simulink model "px42LoopCtr20210902"  (R2022a)
settings: Solver=FixedStepDiscrete  StartTime=0.0  StopTime=inf  FixedStep=0.005  RelTol=1e-3  EnableMultiTasking=on
InitFcn:
  | I_x = 0.00478;
  | I_y = 0.00502;
  | I_z = 0.00736;
  | m=1;
  | L=0.11667;
undefined symbols (not defined in the file): dev, DiscIntNeverNeededParam, Main, pwm_output0
libraries: simulink x30, px4lib x3, px4uORBlib x2, sharedtransform x1
(part 2 of 3)

== system px42LoopCtr20210902/Attitude controller/Subsystem6 ==
  roll : Inport
  roll_des : Inport  Port=2
  Add : Sum  Inputs=+----
  Add1 : Sum  Inputs=+-
  Add2 : Sum  Inputs=+-
  Constant1 : Constant  Value=0
  Data Store Read : DataStoreRead  DataStoreName=attitude_flag  IndexOptions=Index vector (dialog)  Indices=1  OutputSizes=1
  Data Store Read1 : DataStoreRead  DataStoreName=roll_speed  IndexOptions=Index vector (dialog)  Indices=1  OutputSizes=1
  Data Store Write : DataStoreWrite  DataStoreName=e_pitch_roll  IndexOptions=Index vector (dialog)  Indices=1  OutputSizes=1
  Demux : Demux  Outputs=3
  Discrete Derivative1 : simulink/Discrete/Discrete Derivative  gainval=1.0  ICPrevScaledInput=0.0  OutMin=[]  OutMax=[]  OutDataType=fixdt(1, 16)  OutScaling=2^-10  DoSatur=off
  Gain : Gain  Gain=0.01/0.0052
  J : Gain  Gain=0.00478
  Mux : Mux  Inputs=3
  Product : Product  Inputs=3
  Product1 : Product
  Sign : Signum
  Slider : SliderBlock  ScaleMax=20
  Slider1 : SliderBlock  ScaleMax=20
  Slider2 : SliderBlock  ScaleMin=2  ScaleMax=10
  Slider3 : SliderBlock  ScaleMax=20
  Slider4 : SliderBlock  ScaleMax=10
  Subsystem1 : Subsystem
  Switch : Switch  Criteria=u2 > Threshold  SaturateOnIntegerOverflow=off  InputSameDT=off
  b : Constant  Value=2.490277777777778
  l : Constant  Value=0.5340277777777778
  u2 : Outport
  wires:
  Data Store Read1/1 -> Mux/3
  Demux/2 -> Add2/2, Subsystem1/2(roll_des)
  Demux/1 -> Add2/1, Subsystem1/1(roll)
  Mux/1 -> Switch/1
  Constant1/1 -> Switch/3
  Switch/1 -> Demux/1
  Data Store Read/1 -> Switch/2
  Add/1 -> J/1
  Gain/1 -> Add/5
  Product1/1 -> Add/4
  Add2/1 -> Add/2, Data Store Write/1
  roll_des/1 -> Mux/2
  Sign/1 -> Product1/1
  Subsystem1/1(v*) -> Discrete Derivative1/1, Add1/2
  Subsystem1/2(H) -> Product/2
  b/1 -> Product/3, Subsystem1/3(b)
  l/1 -> Product1/2
  Discrete Derivative1/1 -> Add/1  "v*_dot"
  roll/1 -> Mux/1
  Demux/3 -> Add1/1, Gain/1  "v"
  Add1/1 -> Product/1, Sign/1  "v-v*"
  Product/1 -> Add/3
  J/1 -> u2/1

== system px42LoopCtr20210902/Attitude controller/Subsystem7 ==
  yaw : Inport
  yaw_des : Inport  Port=2
  Add : Sum  Inputs=+----
  Add1 : Sum  Inputs=+-
  Add2 : Sum  Inputs=+-
  Constant1 : Constant  Value=0
  Data Store Read : DataStoreRead  DataStoreName=attitude_flag  IndexOptions=Index vector (dialog)  Indices=1  OutputSizes=1
  Data Store Read1 : DataStoreRead  DataStoreName=yaw_speed  IndexOptions=Index vector (dialog)  Indices=1  OutputSizes=1
  Data Store Write : DataStoreWrite  DataStoreName=e_pitch_yaw  IndexOptions=Index vector (dialog)  Indices=1  OutputSizes=1
  Demux : Demux  Outputs=3
  Discrete Derivative1 : simulink/Discrete/Discrete Derivative  gainval=1.0  ICPrevScaledInput=0.0  OutMin=[]  OutMax=[]  OutDataType=fixdt(1, 16)  OutScaling=2^-10  DoSatur=off
  Gain : Gain  Gain=0.01/0.0052
  Gain1 : Gain  Gain=0.00502
  Mux : Mux  Inputs=3
  Product : Product  Inputs=3
  Product1 : Product
  Sign : Signum
  Slider : SliderBlock  ScaleMax=20
  Slider1 : SliderBlock  ScaleMax=20
  Slider2 : SliderBlock  ScaleMin=2  ScaleMax=10
  Slider3 : SliderBlock  ScaleMax=20
  Slider4 : SliderBlock  ScaleMax=10
  Subsystem1 : Subsystem
  Switch : Switch  Criteria=u2 > Threshold  SaturateOnIntegerOverflow=off  InputSameDT=off
  b : Constant  Value=2.036184210526316
  l : Constant  Value=0.5282118055555556
  u2 : Outport
  wires:
  Data Store Read1/1 -> Mux/3
  Demux/2 -> Add2/2, Subsystem1/2(pitch_des)
  Demux/1 -> Add2/1, Subsystem1/1(pitch)
  Mux/1 -> Switch/1
  Constant1/1 -> Switch/3
  Switch/1 -> Demux/1
  Data Store Read/1 -> Switch/2
  Gain1/1 -> u2/1
  Gain/1 -> Add/5
  Product1/1 -> Add/4
  Add2/1 -> Add/2, Data Store Write/1
  yaw_des/1 -> Mux/2
  Add/1 -> Gain1/1
  Sign/1 -> Product1/1
  Subsystem1/1(v*) -> Discrete Derivative1/1, Add1/2
  Subsystem1/2(H) -> Product/2
  b/1 -> Product/3, Subsystem1/3(b)
  l/1 -> Product1/2
  Discrete Derivative1/1 -> Add/1  "v*_dot"
  yaw/1 -> Mux/1
  Demux/3 -> Add1/1, Gain/1  "v"
  Add1/1 -> Product/1, Sign/1  "v-v*"
  Product/1 -> Add/3

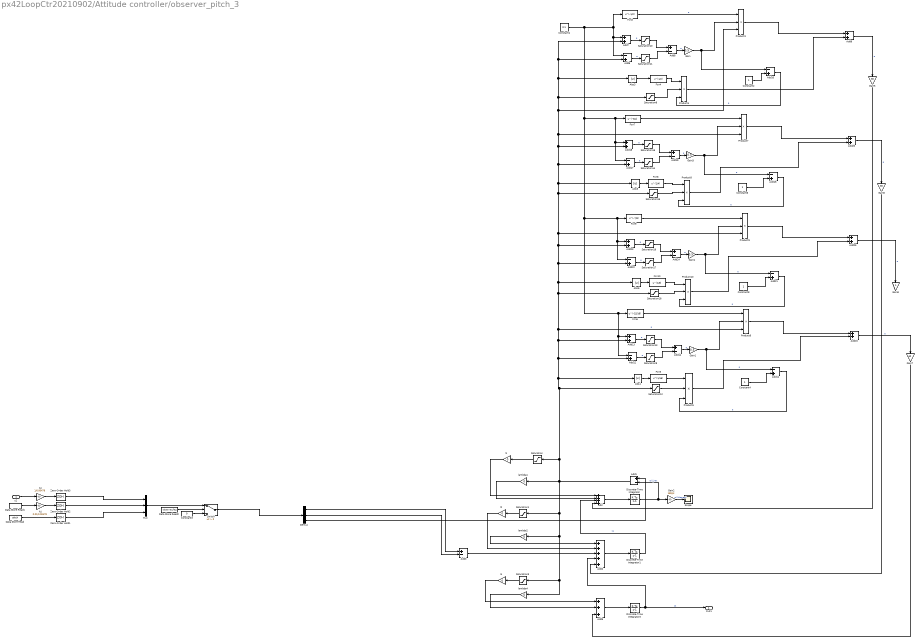
== system px42LoopCtr20210902/Attitude controller/observer_pitch_3 ==
  u2 : Inport
  1/J : Gain  Gain=1/0.00478
  Abs{3..6} (4 alike) : Abs  SaturateOnIntegerOverflow=off
  Add : Sum  Inputs=++++
  Add{1,3,8,14,19,24} (6 alike) : Sum  Inputs=+-
  Add{6,10..12,16..17,21..22} (8 alike) : Sum  Inputs=-+
  Add{7,9,13,15,18,20,23,25} (8 alike) : Sum
  Add2 : Sum  Inputs=+++++
  Add5 : Sum  Inputs=+++
  Constant1 : Constant  Value=0.1
  Constant{2,4,6,8} (4 alike) : Constant
  Constant3 : Constant  Value=0
  Data Store Read : DataStoreRead  DataStoreName=pitch  IndexOptions=Index vector (dialog)  Indices=1  OutputSizes=1
  Data Store Read1 : DataStoreRead  DataStoreName=pitch_speed  IndexOptions=Index vector (dialog)  Indices=1  OutputSizes=1
  Data Store Read2 : DataStoreRead  DataStoreName=observer_flag  IndexOptions=Index vector (dialog)  Indices=1  OutputSizes=1
  Demux : Demux  Outputs=3
  Discrete-Time Integrator : DiscreteIntegrator  SampleTime=-1  ICPrevOutput=DiscIntNeverNeededParam  ICPrevScaledInput=DiscIntNeverNeededParam
  Discrete-Time Integrator1 : DiscreteIntegrator  SampleTime=-1  ICPrevOutput=DiscIntNeverNeededParam  ICPrevScaledInput=DiscIntNeverNeededParam
  Discrete-Time Integrator3 : DiscreteIntegrator  SampleTime=-1  ICPrevOutput=DiscIntNeverNeededParam  ICPrevScaledInput=DiscIntNeverNeededParam
  Fcn10 : Fcn  Expr=u^(1/8)
  Fcn3 : Fcn  Expr=u^(-1/2)
  Fcn4 : Fcn  Expr=u^(1/2)
  Fcn5 : Fcn  Expr=u^(1/16)
  Fcn6 : Fcn  Expr=u^(-15/16)
  Fcn7 : Fcn  Expr=u^(-3/4)
  Fcn8 : Fcn  Expr=u^(1/4)
  Fcn9 : Fcn  Expr=u^(-7/8)
  Gain{,1,3..4} (4 alike) : Gain  Gain=0.5
  Gain2 : Gain  Gain=180/pi
  Gain5 : Gain  Gain=30
  Gain6 : Gain  Gain=30
  Gain7 : Gain  Gain=40
  Gain8 : Gain
  Mux : Mux  Inputs=3
  Product{3..10} (8 alike) : Product  Inputs=3
  Saturation{,1,3,8..19} (15 alike) : Saturate  UpperLimit=1  LowerLimit=-1
  Scope : Scope
  Switch : Switch  Criteria=u2 > Threshold  SaturateOnIntegerOverflow=off  InputSameDT=off
  Zero-Order Hold1 : ZeroOrderHold  SampleTime=-1
  Zero-Order Hold2 : ZeroOrderHold  SampleTime=-1
  Zero-Order Hold3 : ZeroOrderHold  SampleTime=-1
  k/J : Gain  Gain=0.01/0.00478
  l1 : Gain  Gain=0
  l2 : Gain  Gain=0
  l4 : Gain  Gain=0
  lambda1 : Gain  Gain=0
  lambda2 : Gain  Gain=0
  lambda4 : Gain  Gain=0
  Out1 : Outport
  wires:
  Fcn4/1 -> Product4/1
  Fcn3/1 -> Product3/1  "e"
  Gain7/1 -> Add5/3
  Gain6/1 -> Add2/5
  Gain5/1 -> Add/4
  Add9/1 -> Gain5/1  "e"
  Add20/1 -> Gain6/1  "e"
  Add25/1 -> Gain8/1  "e"
  Add15/1 -> Gain7/1  "e"
  Saturation13/1 -> Add14/1
  Add1/1 -> Saturation1/1, lambda2/1, Saturation3/1, lambda4/1, Saturation/1, Saturation15/1, Abs5/1, Add17/2, Add18/2, Abs3/1, Add7/2, Add6/2, Saturation8/1, Product3/3, Product7/3, Product9/3, Add23/2, Add22/2, Abs6/1, Saturation18/1, Product6/3, Add13/2, Add12/2, Abs4/1, Saturation12/1, lambda1/1  "e"
  Add11/1 -> Product5/3  "e"
  Add12/1 -> Saturation9/1  "e"
  Abs4/1 -> Fcn5/1
  Constant4/1 -> Add11/2
  Product6/1 -> Add15/1
  Saturation12/1 -> Product5/2
  Gain1/1 -> Product6/2, Add11/1  "e"
  Add13/1 -> Saturation13/1  "e"
  Fcn6/1 -> Product6/1
  Fcn5/1 -> Product5/1
  Saturation9/1 -> Add14/2
  Product5/1 -> Add15/2
  Constant1/1 -> Fcn9/1, Add23/1, Add22/1, Add13/1, Add12/1, Fcn6/1, Add18/1, Add17/1, Fcn7/1, Add7/1, Add6/1, Fcn3/1
  Add14/1 -> Gain1/1  "e"
  Add24/1 -> Gain4/1  "e"
  Saturation17/1 -> Add24/2
  Product10/1 -> Add25/2
  Fcn10/1 -> Product10/1
  Fcn9/1 -> Product9/1
  Add23/1 -> Saturation19/1  "e"
  Gain4/1 -> Product9/2, Add21/1  "e"
  Saturation18/1 -> Product10/2
  Saturation19/1 -> Add24/1
  Abs6/1 -> Fcn10/1
  Add21/1 -> Product10/3  "e"
  Product9/1 -> Add25/1
  Add22/1 -> Saturation17/1  "e"
  Constant8/1 -> Add21/2
  Product7/1 -> Add20/1
  Saturation15/1 -> Product8/2
  Add17/1 -> Saturation14/1  "e"
  Constant6/1 -> Add16/2
  Gain3/1 -> Product7/2, Add16/1  "e"
  Abs5/1 -> Fcn8/1
  Add16/1 -> Product8/3  "e"
  Saturation16/1 -> Add19/1
  Fcn8/1 -> Product8/1
  Fcn7/1 -> Product7/1
  Product8/1 -> Add20/2
  Add19/1 -> Gain3/1  "e"
  Saturation14/1 -> Add19/2
  Add18/1 -> Saturation16/1  "e"
  Product4/1 -> Add9/2
  Saturation11/1 -> Add8/2
  Saturation10/1 -> Add8/1
  Add10/1 -> Product4/3  "e"
  Constant2/1 -> Add10/2
  Saturation8/1 -> Product4/2
  Abs3/1 -> Fcn4/1
  Product3/1 -> Add9/1
  Gain/1 -> Product3/2, Add10/1
  Add8/1 -> Gain/1  "e"
  Add6/1 -> Saturation11/1  "e"
  Add7/1 -> Saturation10/1  "e"
  Gain2/1 -> Scope/1  "roll(degree)"
  l4/1 -> Add5/1
  lambda4/1 -> Add5/2
  Add5/1 -> Discrete-Time Integrator3/1
  Saturation3/1 -> l4/1
  Add2/1 -> Discrete-Time Integrator1/1
  Add3/1 -> Add2/3
  l2/1 -> Add2/2
  lambda2/1 -> Add2/1
  Saturation1/1 -> l2/1
  Discrete-Time Integrator3/1 -> Out1/1, Add2/4  "z2"
  l1/1 -> Add/1
  Saturation/1 -> l1/1
  lambda1/1 -> Add/2
  Discrete-Time Integrator/1 -> Gain2/1, Add1/2  "roll_hat"
  Discrete-Time Integrator1/1 -> Add/3  "z1"
  Add/1 -> Discrete-Time Integrator/1
  Demux/1 -> Add3/1
  Demux/2 -> Add3/2
  Demux/3 -> Add1/1
  k/J/1 -> Zero-Order Hold2/1
  Data Store Read1/1 -> k/J/1
  Zero-Order Hold2/1 -> Mux/2
  Mux/1 -> Switch/1
  Zero-Order Hold3/1 -> Mux/1
  u2/1 -> 1/J/1
  Switch/1 -> Demux/1
  Data Store Read2/1 -> Switch/2
  Zero-Order Hold1/1 -> Mux/3
  Data Store Read/1 -> Zero-Order Hold1/1
  1/J/1 -> Zero-Order Hold3/1
  Constant3/1 -> Switch/3

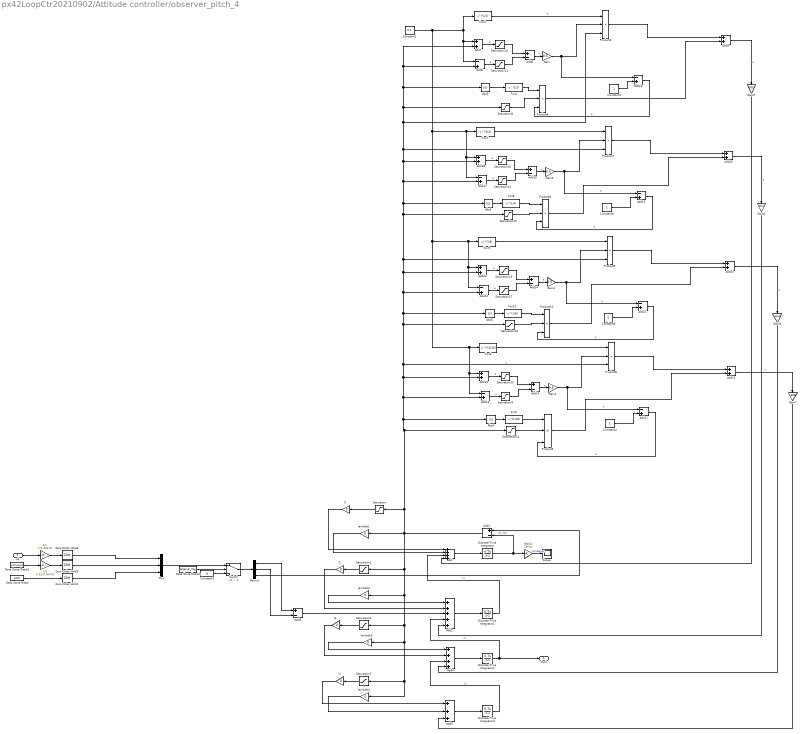
== system px42LoopCtr20210902/Attitude controller/observer_pitch_4 ==
  u2 : Inport
  1/J : Gain  Gain=1/0.00478
  Abs{3..6} (4 alike) : Abs  SaturateOnIntegerOverflow=off
  Add : Sum  Inputs=++++
  Add{1,3,8,14,19,24} (6 alike) : Sum  Inputs=+-
  Add{6,10..12,16..17,21..22} (8 alike) : Sum  Inputs=-+
  Add{7,9,13,15,18,20,23,25} (8 alike) : Sum
  Add2 : Sum  Inputs=+++++
  Add4 : Sum  Inputs=++++
  Add5 : Sum  Inputs=+++
  Constant1 : Constant  Value=0.1
  Constant{2,4,6,8} (4 alike) : Constant
  Constant3 : Constant  Value=0
  Data Store Read : DataStoreRead  DataStoreName=pitch  IndexOptions=Index vector (dialog)  Indices=1  OutputSizes=1
  Data Store Read1 : DataStoreRead  DataStoreName=pitch_speed  IndexOptions=Index vector (dialog)  Indices=1  OutputSizes=1
  Data Store Read2 : DataStoreRead  DataStoreName=observer_flag  IndexOptions=Index vector (dialog)  Indices=1  OutputSizes=1
  Demux : Demux  Outputs=3
  Discrete-Time Integrator{,1..3} (4 alike) : DiscreteIntegrator  SampleTime=-1  ICPrevOutput=DiscIntNeverNeededParam  ICPrevScaledInput=DiscIntNeverNeededParam
  Fcn10 : Fcn  Expr=u^(1/8)
  Fcn3 : Fcn  Expr=u^(-1/2)
  Fcn4 : Fcn  Expr=u^(1/2)
  Fcn5 : Fcn  Expr=u^(1/16)
  Fcn6 : Fcn  Expr=u^(-15/16)
  Fcn7 : Fcn  Expr=u^(-3/4)
  Fcn8 : Fcn  Expr=u^(1/4)
  Fcn9 : Fcn  Expr=u^(-7/8)
  Gain{,1,3..4} (4 alike) : Gain  Gain=0.5
  Gain2 : Gain  Gain=180/pi
  Gain5 : Gain  Gain=300
  Gain6 : Gain  Gain=3000
  Gain7 : Gain  Gain=300
  Gain8 : Gain  Gain=5000
  Mux : Mux  Inputs=3
  Product{3..10} (8 alike) : Product  Inputs=3
  Saturation{,1..3,8..19} (16 alike) : Saturate  UpperLimit=1  LowerLimit=-1
  Scope : Scope
  Switch : Switch  Criteria=u2 > Threshold  SaturateOnIntegerOverflow=off  InputSameDT=off
  Zero-Order Hold1 : ZeroOrderHold  SampleTime=-1
  Zero-Order Hold2 : ZeroOrderHold  SampleTime=-1
  Zero-Order Hold3 : ZeroOrderHold  SampleTime=-1
  k/J : Gain  Gain=0.01/0.00478
  l{1..4} (4 alike) : Gain  Gain=0
  lambda{1..4} (4 alike) : Gain  Gain=0
  Out1 : Outport
  wires:
  Zero-Order Hold1/1 -> Mux/3
  Demux/3 -> Add1/1
  Demux/2 -> Add3/2
  Demux/1 -> Add3/1
  Zero-Order Hold3/1 -> Mux/1
  Mux/1 -> Switch/1
  Constant3/1 -> Switch/3
  Zero-Order Hold2/1 -> Mux/2
  Switch/1 -> Demux/1
  Add/1 -> Discrete-Time Integrator/1
  Discrete-Time Integrator1/1 -> Add/3  "z1"
  Discrete-Time Integrator/1 -> Add1/2, Gain2/1  "roll_hat"
  Data Store Read/1 -> Zero-Order Hold1/1
  lambda1/1 -> Add/2
  Saturation/1 -> l1/1
  l1/1 -> Add/1
  Discrete-Time Integrator2/1 -> Out1/1, Add2/4  "z2"
  Saturation1/1 -> l2/1
  lambda2/1 -> Add2/1
  l2/1 -> Add2/2
  Data Store Read1/1 -> k/J/1
  k/J/1 -> Zero-Order Hold2/1
  u2/1 -> 1/J/1
  1/J/1 -> Zero-Order Hold3/1
  Add3/1 -> Add2/3
  Add2/1 -> Discrete-Time Integrator1/1
  Discrete-Time Integrator3/1 -> Add4/3  "z3"
  Add4/1 -> Discrete-Time Integrator2/1
  Saturation2/1 -> l3/1
  lambda3/1 -> Add4/1
  l3/1 -> Add4/2
  Saturation3/1 -> l4/1
  Add5/1 -> Discrete-Time Integrator3/1
  lambda4/1 -> Add5/2
  l4/1 -> Add5/1
  Gain2/1 -> Scope/1  "roll(degree)"
  Add7/1 -> Saturation10/1  "e"
  Add6/1 -> Saturation11/1  "e"
  Add8/1 -> Gain/1  "e"
  Gain/1 -> Add10/1, Product3/2
  Product3/1 -> Add9/1
  Abs3/1 -> Fcn4/1
  Saturation8/1 -> Product4/2
  Constant2/1 -> Add10/2
  Add10/1 -> Product4/3  "e"
  Saturation10/1 -> Add8/1
  Saturation11/1 -> Add8/2
  Product4/1 -> Add9/2
  Add18/1 -> Saturation16/1  "e"
  Saturation14/1 -> Add19/2
  Add19/1 -> Gain3/1  "e"
  Product8/1 -> Add20/2
  Fcn7/1 -> Product7/1
  Fcn8/1 -> Product8/1
  Saturation16/1 -> Add19/1
  Add16/1 -> Product8/3  "e"
  Abs5/1 -> Fcn8/1
  Gain3/1 -> Add16/1, Product7/2  "e"
  Constant6/1 -> Add16/2
  Add17/1 -> Saturation14/1  "e"
  Saturation15/1 -> Product8/2
  Product7/1 -> Add20/1
  Constant8/1 -> Add21/2
  Add22/1 -> Saturation17/1  "e"
  Product9/1 -> Add25/1
  Add21/1 -> Product10/3  "e"
  Abs6/1 -> Fcn10/1
  Saturation19/1 -> Add24/1
  Saturation18/1 -> Product10/2
  Gain4/1 -> Add21/1, Product9/2  "e"
  Add23/1 -> Saturation19/1  "e"
  Fcn9/1 -> Product9/1
  Fcn10/1 -> Product10/1
  Product10/1 -> Add25/2
  Saturation17/1 -> Add24/2
  Add24/1 -> Gain4/1  "e"
  Add14/1 -> Gain1/1  "e"
  Constant1/1 -> Fcn3/1, Add6/1, Add7/1, Fcn7/1, Add17/1, Add18/1, Fcn6/1, Add12/1, Add13/1, Add22/1, Add23/1, Fcn9/1
  Product5/1 -> Add15/2
  Saturation9/1 -> Add14/2
  Fcn5/1 -> Product5/1
  Fcn6/1 -> Product6/1
  Add13/1 -> Saturation13/1  "e"
  Gain1/1 -> Add11/1, Product6/2  "e"
  Saturation12/1 -> Product5/2
  Product6/1 -> Add15/1
  Constant4/1 -> Add11/2
  Abs4/1 -> Fcn5/1
  Add12/1 -> Saturation9/1  "e"
  Add11/1 -> Product5/3  "e"
  Add1/1 -> lambda1/1, Saturation12/1, Abs4/1, Add12/2, Add13/2, Product6/3, Saturation18/1, Abs6/1, Add22/2, Add23/2, Product9/3, Product7/3, Product3/3, Saturation8/1, Add6/2, Add7/2, Abs3/1, Add18/2, Add17/2, Abs5/1, Saturation15/1, Saturation/1, lambda4/1, Saturation3/1, lambda3/1, Saturation2/1, lambda2/1, Saturation1/1  "e"
  Saturation13/1 -> Add14/1
  Add15/1 -> Gain7/1  "e"
  Add25/1 -> Gain8/1  "e"
  Add20/1 -> Gain6/1  "e"
  Add9/1 -> Gain5/1  "e"
  Gain5/1 -> Add/4
  Gain6/1 -> Add2/5
  Gain7/1 -> Add5/3
  Gain8/1 -> Add4/4
  Fcn3/1 -> Product3/1  "e"
  Fcn4/1 -> Product4/1
  Data Store Read2/1 -> Switch/2

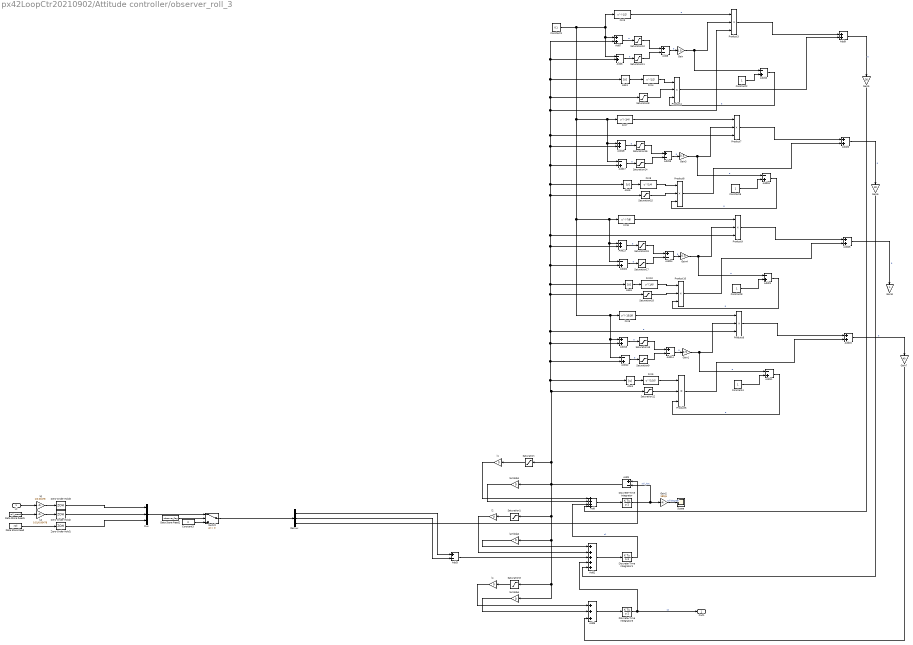
== system px42LoopCtr20210902/Attitude controller/observer_roll_3 ==
  u2 : Inport
  1/J : Gain  Gain=1/0.00478
  Abs{3..6} (4 alike) : Abs  SaturateOnIntegerOverflow=off
  Add : Sum  Inputs=++++
  Add{1,3,8,14,19,24} (6 alike) : Sum  Inputs=+-
  Add{6,10..12,16..17,21..22} (8 alike) : Sum  Inputs=-+
  Add{7,9,13,15,18,20,23,25} (8 alike) : Sum
  Add2 : Sum  Inputs=+++++
  Add5 : Sum  Inputs=+++
  Constant1 : Constant  Value=0.1
  Constant{2,4,6,8} (4 alike) : Constant
  Constant3 : Constant  Value=0
  Data Store Read : DataStoreRead  DataStoreName=roll  IndexOptions=Index vector (dialog)  Indices=1  OutputSizes=1
  Data Store Read1 : DataStoreRead  DataStoreName=roll_speed  IndexOptions=Index vector (dialog)  Indices=1  OutputSizes=1
  Data Store Read2 : DataStoreRead  DataStoreName=observer_flag  IndexOptions=Index vector (dialog)  Indices=1  OutputSizes=1
  Demux : Demux  Outputs=3
  Discrete-Time Integrator : DiscreteIntegrator  SampleTime=-1  ICPrevOutput=DiscIntNeverNeededParam  ICPrevScaledInput=DiscIntNeverNeededParam
  Discrete-Time Integrator1 : DiscreteIntegrator  SampleTime=-1  ICPrevOutput=DiscIntNeverNeededParam  ICPrevScaledInput=DiscIntNeverNeededParam
  Discrete-Time Integrator3 : DiscreteIntegrator  SampleTime=-1  ICPrevOutput=DiscIntNeverNeededParam  ICPrevScaledInput=DiscIntNeverNeededParam
  Fcn10 : Fcn  Expr=u^(1/8)
  Fcn3 : Fcn  Expr=u^(-1/2)
  Fcn4 : Fcn  Expr=u^(1/2)
  Fcn5 : Fcn  Expr=u^(1/16)
  Fcn6 : Fcn  Expr=u^(-15/16)
  Fcn7 : Fcn  Expr=u^(-3/4)
  Fcn8 : Fcn  Expr=u^(1/4)
  Fcn9 : Fcn  Expr=u^(-7/8)
  Gain{,1,3..4} (4 alike) : Gain  Gain=0.5
  Gain2 : Gain  Gain=180/pi
  Gain5 : Gain  Gain=30
  Gain6 : Gain  Gain=30
  Gain7 : Gain  Gain=40
  Gain8 : Gain
  Mux : Mux  Inputs=3
  Product{3..10} (8 alike) : Product  Inputs=3
  Saturation{,1,3,8..19} (15 alike) : Saturate  UpperLimit=1  LowerLimit=-1
  Scope : Scope
  Switch : Switch  Criteria=u2 > Threshold  SaturateOnIntegerOverflow=off  InputSameDT=off
  Zero-Order Hold1 : ZeroOrderHold  SampleTime=-1
  Zero-Order Hold2 : ZeroOrderHold  SampleTime=-1
  Zero-Order Hold3 : ZeroOrderHold  SampleTime=-1
  k/J : Gain  Gain=0.01/0.00478
  l1 : Gain  Gain=0
  l2 : Gain  Gain=0
  l4 : Gain  Gain=0
  lambda1 : Gain  Gain=0
  lambda2 : Gain  Gain=0
  lambda4 : Gain  Gain=0
  Out1 : Outport
  wires:
  Demux/3 -> Add1/1
  Demux/2 -> Add3/2
  Demux/1 -> Add3/1
  Add/1 -> Discrete-Time Integrator/1
  Discrete-Time Integrator1/1 -> Add/3  "z1"
  Discrete-Time Integrator/1 -> Add1/2, Gain2/1  "roll_hat"
  lambda1/1 -> Add/2
  Saturation/1 -> l1/1
  l1/1 -> Add/1
  Discrete-Time Integrator3/1 -> Add2/4, Out1/1  "z2"
  Saturation1/1 -> l2/1
  lambda2/1 -> Add2/1
  l2/1 -> Add2/2
  Add3/1 -> Add2/3
  Add2/1 -> Discrete-Time Integrator1/1
  Saturation3/1 -> l4/1
  Add5/1 -> Discrete-Time Integrator3/1
  lambda4/1 -> Add5/2
  l4/1 -> Add5/1
  Gain2/1 -> Scope/1  "roll(degree)"
  Add7/1 -> Saturation10/1  "e"
  Add6/1 -> Saturation11/1  "e"
  Add8/1 -> Gain/1  "e"
  Gain/1 -> Add10/1, Product3/2
  Product3/1 -> Add9/1
  Abs3/1 -> Fcn4/1
  Saturation8/1 -> Product4/2
  Constant2/1 -> Add10/2
  Add10/1 -> Product4/3  "e"
  Saturation10/1 -> Add8/1
  Saturation11/1 -> Add8/2
  Product4/1 -> Add9/2
  Add18/1 -> Saturation16/1  "e"
  Saturation14/1 -> Add19/2
  Add19/1 -> Gain3/1  "e"
  Product8/1 -> Add20/2
  Fcn7/1 -> Product7/1
  Fcn8/1 -> Product8/1
  Saturation16/1 -> Add19/1
  Add16/1 -> Product8/3  "e"
  Abs5/1 -> Fcn8/1
  Gain3/1 -> Add16/1, Product7/2  "e"
  Constant6/1 -> Add16/2
  Add17/1 -> Saturation14/1  "e"
  Saturation15/1 -> Product8/2
  Product7/1 -> Add20/1
  Constant8/1 -> Add21/2
  Add22/1 -> Saturation17/1  "e"
  Product9/1 -> Add25/1
  Add21/1 -> Product10/3  "e"
  Abs6/1 -> Fcn10/1
  Saturation19/1 -> Add24/1
  Saturation18/1 -> Product10/2
  Gain4/1 -> Add21/1, Product9/2  "e"
  Add23/1 -> Saturation19/1  "e"
  Fcn9/1 -> Product9/1
  Fcn10/1 -> Product10/1
  Product10/1 -> Add25/2
  Saturation17/1 -> Add24/2
  Add24/1 -> Gain4/1  "e"
  Add14/1 -> Gain1/1  "e"
  Constant1/1 -> Fcn3/1, Add6/1, Add7/1, Fcn7/1, Add17/1, Add18/1, Fcn6/1, Add12/1, Add13/1, Add22/1, Add23/1, Fcn9/1
  Product5/1 -> Add15/2
  Saturation9/1 -> Add14/2
  Fcn5/1 -> Product5/1
  Fcn6/1 -> Product6/1
  Add13/1 -> Saturation13/1  "e"
  Gain1/1 -> Add11/1, Product6/2  "e"
  Saturation12/1 -> Product5/2
  Product6/1 -> Add15/1
  Constant4/1 -> Add11/2
  Abs4/1 -> Fcn5/1
  Add12/1 -> Saturation9/1  "e"
  Add11/1 -> Product5/3  "e"
  Add1/1 -> lambda1/1, Saturation12/1, Abs4/1, Add12/2, Add13/2, Product6/3, Saturation18/1, Abs6/1, Add22/2, Add23/2, Product9/3, Product7/3, Product3/3, Saturation8/1, Add6/2, Add7/2, Abs3/1, Add18/2, Add17/2, Abs5/1, Saturation15/1, Saturation/1, lambda4/1, Saturation3/1, lambda2/1, Saturation1/1  "e"
  Saturation13/1 -> Add14/1
  Add15/1 -> Gain7/1  "e"
  Add25/1 -> Gain8/1  "e"
  Add20/1 -> Gain6/1  "e"
  Add9/1 -> Gain5/1  "e"
  Gain5/1 -> Add/4
  Gain6/1 -> Add2/5
  Gain7/1 -> Add5/3
  Fcn3/1 -> Product3/1  "e"
  Fcn4/1 -> Product4/1
  Constant3/1 -> Switch/3
  u2/1 -> 1/J/1
  Zero-Order Hold1/1 -> Mux/3
  Zero-Order Hold2/1 -> Mux/2
  Zero-Order Hold3/1 -> Mux/1
  Data Store Read/1 -> Zero-Order Hold1/1
  Switch/1 -> Demux/1
  Data Store Read2/1 -> Switch/2
  Data Store Read1/1 -> k/J/1
  1/J/1 -> Zero-Order Hold3/1
  Mux/1 -> Switch/1
  k/J/1 -> Zero-Order Hold2/1

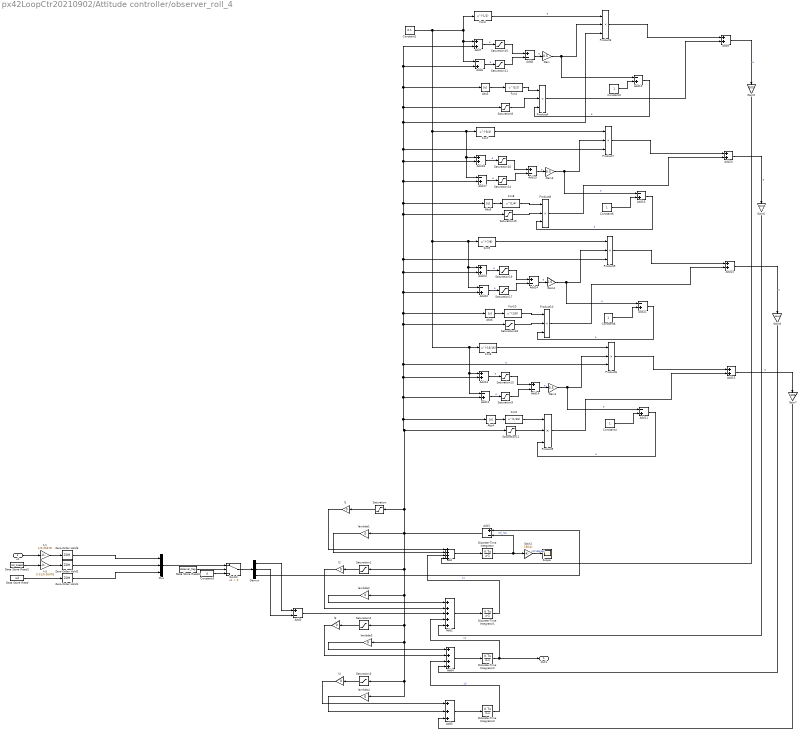
== system px42LoopCtr20210902/Attitude controller/observer_roll_4 ==
  u2 : Inport
  1/J : Gain  Gain=1/0.00478
  Abs{3..6} (4 alike) : Abs  SaturateOnIntegerOverflow=off
  Add : Sum  Inputs=++++
  Add{1,3,8,14,19,24} (6 alike) : Sum  Inputs=+-
  Add{6,10..12,16..17,21..22} (8 alike) : Sum  Inputs=-+
  Add{7,9,13,15,18,20,23,25} (8 alike) : Sum
  Add2 : Sum  Inputs=+++++
  Add4 : Sum  Inputs=++++
  Add5 : Sum  Inputs=+++
  Constant1 : Constant  Value=0.1
  Constant{2,4,6,8} (4 alike) : Constant
  Constant3 : Constant  Value=0
  Data Store Read : DataStoreRead  DataStoreName=roll  IndexOptions=Index vector (dialog)  Indices=1  OutputSizes=1
  Data Store Read1 : DataStoreRead  DataStoreName=roll_speed  IndexOptions=Index vector (dialog)  Indices=1  OutputSizes=1
  Data Store Read2 : DataStoreRead  DataStoreName=observer_flag  IndexOptions=Index vector (dialog)  Indices=1  OutputSizes=1
  Demux : Demux  Outputs=3
  Discrete-Time Integrator{,1..3} (4 alike) : DiscreteIntegrator  SampleTime=-1  ICPrevOutput=DiscIntNeverNeededParam  ICPrevScaledInput=DiscIntNeverNeededParam
  Fcn10 : Fcn  Expr=u^(1/8)
  Fcn3 : Fcn  Expr=u^(-1/2)
  Fcn4 : Fcn  Expr=u^(1/2)
  Fcn5 : Fcn  Expr=u^(1/16)
  Fcn6 : Fcn  Expr=u^(-15/16)
  Fcn7 : Fcn  Expr=u^(-3/4)
  Fcn8 : Fcn  Expr=u^(1/4)
  Fcn9 : Fcn  Expr=u^(-7/8)
  Gain{,1,3..4} (4 alike) : Gain  Gain=0.5
  Gain2 : Gain  Gain=180/pi
  Gain5 : Gain  Gain=300
  Gain6 : Gain  Gain=3000
  Gain7 : Gain  Gain=300
  Gain8 : Gain  Gain=5000
  Mux : Mux  Inputs=3
  Product{3..10} (8 alike) : Product  Inputs=3
  Saturation{,1..3,8..19} (16 alike) : Saturate  UpperLimit=1  LowerLimit=-1
  Scope : Scope
  Switch : Switch  Criteria=u2 > Threshold  SaturateOnIntegerOverflow=off  InputSameDT=off
  Zero-Order Hold1 : ZeroOrderHold  SampleTime=-1
  Zero-Order Hold2 : ZeroOrderHold  SampleTime=-1
  Zero-Order Hold3 : ZeroOrderHold  SampleTime=-1
  k/J : Gain  Gain=0.01/0.00478
  l{1..4} (4 alike) : Gain  Gain=0
  lambda{1..4} (4 alike) : Gain  Gain=0
  Out1 : Outport
  wires:
  Fcn4/1 -> Product4/1
  Fcn3/1 -> Product3/1  "e"
  Gain8/1 -> Add4/4
  Gain7/1 -> Add5/3
  Gain6/1 -> Add2/5
  Gain5/1 -> Add/4
  Add9/1 -> Gain5/1  "e"
  Add20/1 -> Gain6/1  "e"
  Add25/1 -> Gain8/1  "e"
  Add15/1 -> Gain7/1  "e"
  Saturation13/1 -> Add14/1
  Add1/1 -> Saturation1/1, lambda2/1, Saturation2/1, lambda3/1, Saturation3/1, lambda4/1, Saturation/1, Saturation15/1, Abs5/1, Add17/2, Add18/2, Abs3/1, Add7/2, Add6/2, Saturation8/1, Product3/3, Product7/3, Product9/3, Add23/2, Add22/2, Abs6/1, Saturation18/1, Product6/3, Add13/2, Add12/2, Abs4/1, Saturation12/1, lambda1/1  "e"
  Add11/1 -> Product5/3  "e"
  Add12/1 -> Saturation9/1  "e"
  Abs4/1 -> Fcn5/1
  Constant4/1 -> Add11/2
  Product6/1 -> Add15/1
  Saturation12/1 -> Product5/2
  Gain1/1 -> Product6/2, Add11/1  "e"
  Add13/1 -> Saturation13/1  "e"
  Fcn6/1 -> Product6/1
  Fcn5/1 -> Product5/1
  Saturation9/1 -> Add14/2
  Product5/1 -> Add15/2
  Constant1/1 -> Fcn9/1, Add23/1, Add22/1, Add13/1, Add12/1, Fcn6/1, Add18/1, Add17/1, Fcn7/1, Add7/1, Add6/1, Fcn3/1
  Add14/1 -> Gain1/1  "e"
  Add24/1 -> Gain4/1  "e"
  Saturation17/1 -> Add24/2
  Product10/1 -> Add25/2
  Fcn10/1 -> Product10/1
  Fcn9/1 -> Product9/1
  Add23/1 -> Saturation19/1  "e"
  Gain4/1 -> Product9/2, Add21/1  "e"
  Saturation18/1 -> Product10/2
  Saturation19/1 -> Add24/1
  Abs6/1 -> Fcn10/1
  Add21/1 -> Product10/3  "e"
  Product9/1 -> Add25/1
  Add22/1 -> Saturation17/1  "e"
  Constant8/1 -> Add21/2
  Product7/1 -> Add20/1
  Saturation15/1 -> Product8/2
  Add17/1 -> Saturation14/1  "e"
  Constant6/1 -> Add16/2
  Gain3/1 -> Product7/2, Add16/1  "e"
  Abs5/1 -> Fcn8/1
  Add16/1 -> Product8/3  "e"
  Saturation16/1 -> Add19/1
  Fcn8/1 -> Product8/1
  Fcn7/1 -> Product7/1
  Product8/1 -> Add20/2
  Add19/1 -> Gain3/1  "e"
  Saturation14/1 -> Add19/2
  Add18/1 -> Saturation16/1  "e"
  Product4/1 -> Add9/2
  Saturation11/1 -> Add8/2
  Saturation10/1 -> Add8/1
  Add10/1 -> Product4/3  "e"
  Constant2/1 -> Add10/2
  Saturation8/1 -> Product4/2
  Abs3/1 -> Fcn4/1
  Product3/1 -> Add9/1
  Gain/1 -> Product3/2, Add10/1
  Add8/1 -> Gain/1  "e"
  Add6/1 -> Saturation11/1  "e"
  Add7/1 -> Saturation10/1  "e"
  Gain2/1 -> Scope/1  "roll(degree)"
  l4/1 -> Add5/1
  lambda4/1 -> Add5/2
  Add5/1 -> Discrete-Time Integrator3/1
  Saturation3/1 -> l4/1
  l3/1 -> Add4/2
  lambda3/1 -> Add4/1
  Saturation2/1 -> l3/1
  Add4/1 -> Discrete-Time Integrator2/1
  Discrete-Time Integrator3/1 -> Add4/3  "z3"
  Add2/1 -> Discrete-Time Integrator1/1
  Add3/1 -> Add2/3
  1/J/1 -> Zero-Order Hold3/1
  u2/1 -> 1/J/1
  k/J/1 -> Zero-Order Hold2/1
  Data Store Read1/1 -> k/J/1
  l2/1 -> Add2/2
  lambda2/1 -> Add2/1
  Saturation1/1 -> l2/1
  Discrete-Time Integrator2/1 -> Add2/4, Out1/1  "z2"
  l1/1 -> Add/1
  Saturation/1 -> l1/1
  lambda1/1 -> Add/2
  Data Store Read/1 -> Zero-Order Hold1/1
  Discrete-Time Integrator/1 -> Gain2/1, Add1/2  "roll_hat"
  Discrete-Time Integrator1/1 -> Add/3  "z1"
  Add/1 -> Discrete-Time Integrator/1
  Switch/1 -> Demux/1
  Zero-Order Hold2/1 -> Mux/2
  Data Store Read2/1 -> Switch/2
  Constant3/1 -> Switch/3
  Mux/1 -> Switch/1
  Zero-Order Hold3/1 -> Mux/1
  Demux/1 -> Add3/1
  Demux/2 -> Add3/2
  Demux/3 -> Add1/1
  Zero-Order Hold1/1 -> Mux/3

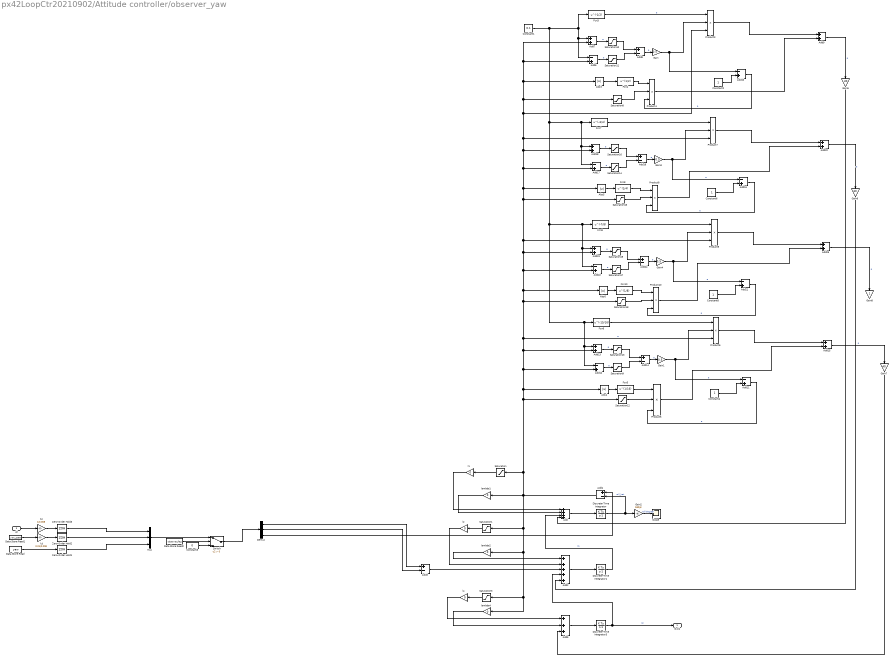
== system px42LoopCtr20210902/Attitude controller/observer_yaw ==
  u2 : Inport
  1/J : Gain  Gain=1/0.008
  Abs{3..6} (4 alike) : Abs  SaturateOnIntegerOverflow=off
  Add : Sum  Inputs=++++
  Add{1,3,8,14,19,24} (6 alike) : Sum  Inputs=+-
  Add{6,10..12,16..17,21..22} (8 alike) : Sum  Inputs=-+
  Add{7,9,13,15,18,20,23,25} (8 alike) : Sum
  Add2 : Sum  Inputs=+++++
  Add5 : Sum  Inputs=+++
  Constant1 : Constant  Value=0.1
  Constant{2,4,6,8} (4 alike) : Constant
  Constant3 : Constant  Value=0
  Data Store Read : DataStoreRead  DataStoreName=yaw  IndexOptions=Index vector (dialog)  Indices=1  OutputSizes=1
  Data Store Read1 : DataStoreRead  DataStoreName=yaw_speed  IndexOptions=Index vector (dialog)  Indices=1  OutputSizes=1
  Data Store Read2 : DataStoreRead  DataStoreName=observer_flag  IndexOptions=Index vector (dialog)  Indices=1  OutputSizes=1
  Demux : Demux  Outputs=3
  Discrete-Time Integrator : DiscreteIntegrator  SampleTime=-1  ICPrevOutput=DiscIntNeverNeededParam  ICPrevScaledInput=DiscIntNeverNeededParam
  Discrete-Time Integrator1 : DiscreteIntegrator  SampleTime=-1  ICPrevOutput=DiscIntNeverNeededParam  ICPrevScaledInput=DiscIntNeverNeededParam
  Discrete-Time Integrator3 : DiscreteIntegrator  SampleTime=-1  ICPrevOutput=DiscIntNeverNeededParam  ICPrevScaledInput=DiscIntNeverNeededParam
  Fcn10 : Fcn  Expr=u^(1/8)
  Fcn3 : Fcn  Expr=u^(-1/2)
  Fcn4 : Fcn  Expr=u^(1/2)
  Fcn5 : Fcn  Expr=u^(1/16)
  Fcn6 : Fcn  Expr=u^(-15/16)
  Fcn7 : Fcn  Expr=u^(-3/4)
  Fcn8 : Fcn  Expr=u^(1/4)
  Fcn9 : Fcn  Expr=u^(-7/8)
  Gain{,1,3..4} (4 alike) : Gain  Gain=0.5
  Gain2 : Gain  Gain=180/pi
  Gain5 : Gain  Gain=30
  Gain6 : Gain  Gain=30
  Gain7 : Gain  Gain=40
  Gain8 : Gain
  Mux : Mux  Inputs=3
  Product{3..10} (8 alike) : Product  Inputs=3
  Saturation{,1,3,8..19} (15 alike) : Saturate  UpperLimit=1  LowerLimit=-1
  Scope : Scope
  Switch : Switch  Criteria=u2 > Threshold  SaturateOnIntegerOverflow=off  InputSameDT=off
  Zero-Order Hold1 : ZeroOrderHold  SampleTime=-1
  Zero-Order Hold2 : ZeroOrderHold  SampleTime=-1
  Zero-Order Hold3 : ZeroOrderHold  SampleTime=-1
  k/J : Gain  Gain=0.01/0.008
  l1 : Gain  Gain=0
  l2 : Gain  Gain=0
  l4 : Gain  Gain=0
  lambda1 : Gain  Gain=0
  lambda2 : Gain  Gain=0
  lambda4 : Gain  Gain=0
  Out1 : Outport
  wires:
  Fcn4/1 -> Product4/1
  Fcn3/1 -> Product3/1  "e"
  Gain7/1 -> Add5/3
  Gain6/1 -> Add2/5
  Gain5/1 -> Add/4
  Add9/1 -> Gain5/1  "e"
  Add20/1 -> Gain6/1  "e"
  Add25/1 -> Gain8/1  "e"
  Add15/1 -> Gain7/1  "e"
  Saturation13/1 -> Add14/1
  Add1/1 -> Saturation1/1, lambda2/1, Saturation3/1, lambda4/1, Saturation/1, Saturation15/1, Abs5/1, Add17/2, Add18/2, Abs3/1, Add7/2, Add6/2, Saturation8/1, Product3/3, Product7/3, Product9/3, Add23/2, Add22/2, Abs6/1, Saturation18/1, Product6/3, Add13/2, Add12/2, Abs4/1, Saturation12/1, lambda1/1  "e"
  Add11/1 -> Product5/3  "e"
  Add12/1 -> Saturation9/1  "e"
  Abs4/1 -> Fcn5/1
  Constant4/1 -> Add11/2
  Product6/1 -> Add15/1
  Saturation12/1 -> Product5/2
  Gain1/1 -> Product6/2, Add11/1  "e"
  Add13/1 -> Saturation13/1  "e"
  Fcn6/1 -> Product6/1
  Fcn5/1 -> Product5/1
  Saturation9/1 -> Add14/2
  Product5/1 -> Add15/2
  Constant1/1 -> Fcn9/1, Add23/1, Add22/1, Add13/1, Add12/1, Fcn6/1, Add18/1, Add17/1, Fcn7/1, Add7/1, Add6/1, Fcn3/1
  Add14/1 -> Gain1/1  "e"
  Add24/1 -> Gain4/1  "e"
  Saturation17/1 -> Add24/2
  Product10/1 -> Add25/2
  Fcn10/1 -> Product10/1
  Fcn9/1 -> Product9/1
  Add23/1 -> Saturation19/1  "e"
  Gain4/1 -> Product9/2, Add21/1  "e"
  Saturation18/1 -> Product10/2
  Saturation19/1 -> Add24/1
  Abs6/1 -> Fcn10/1
  Add21/1 -> Product10/3  "e"
  Product9/1 -> Add25/1
  Add22/1 -> Saturation17/1  "e"
  Constant8/1 -> Add21/2
  Product7/1 -> Add20/1
  Saturation15/1 -> Product8/2
  Add17/1 -> Saturation14/1  "e"
  Constant6/1 -> Add16/2
  Gain3/1 -> Product7/2, Add16/1  "e"
  Abs5/1 -> Fcn8/1
  Add16/1 -> Product8/3  "e"
  Saturation16/1 -> Add19/1
  Fcn8/1 -> Product8/1
  Fcn7/1 -> Product7/1
  Product8/1 -> Add20/2
  Add19/1 -> Gain3/1  "e"
  Saturation14/1 -> Add19/2
  Add18/1 -> Saturation16/1  "e"
  Product4/1 -> Add9/2
  Saturation11/1 -> Add8/2
  Saturation10/1 -> Add8/1
  Add10/1 -> Product4/3  "e"
  Constant2/1 -> Add10/2
  Saturation8/1 -> Product4/2
  Abs3/1 -> Fcn4/1
  Product3/1 -> Add9/1
  Gain/1 -> Product3/2, Add10/1
  Add8/1 -> Gain/1  "e"
  Add6/1 -> Saturation11/1  "e"
  Add7/1 -> Saturation10/1  "e"
  Gain2/1 -> Scope/1  "roll(degree)"
  l4/1 -> Add5/1
  lambda4/1 -> Add5/2
  Add5/1 -> Discrete-Time Integrator3/1
  Saturation3/1 -> l4/1
  Add2/1 -> Discrete-Time Integrator1/1
  Add3/1 -> Add2/3
  l2/1 -> Add2/2
  lambda2/1 -> Add2/1
  Saturation1/1 -> l2/1
  Discrete-Time Integrator3/1 -> Out1/1, Add2/4  "z2"
  l1/1 -> Add/1
  Saturation/1 -> l1/1
  lambda1/1 -> Add/2
  Discrete-Time Integrator/1 -> Gain2/1, Add1/2  "roll_hat"
  Discrete-Time Integrator1/1 -> Add/3  "z1"
  Add/1 -> Discrete-Time Integrator/1
  Demux/1 -> Add3/1
  Demux/2 -> Add3/2
  Demux/3 -> Add1/1
  k/J/1 -> Zero-Order Hold2/1
  Zero-Order Hold1/1 -> Mux/3
  Data Store Read/1 -> Zero-Order Hold1/1
  Constant3/1 -> Switch/3
  Data Store Read2/1 -> Switch/2
  Switch/1 -> Demux/1
  Zero-Order Hold2/1 -> Mux/2
  Zero-Order Hold3/1 -> Mux/1
  Data Store Read1/1 -> k/J/1
  u2/1 -> 1/J/1
  Mux/1 -> Switch/1
  1/J/1 -> Zero-Order Hold3/1

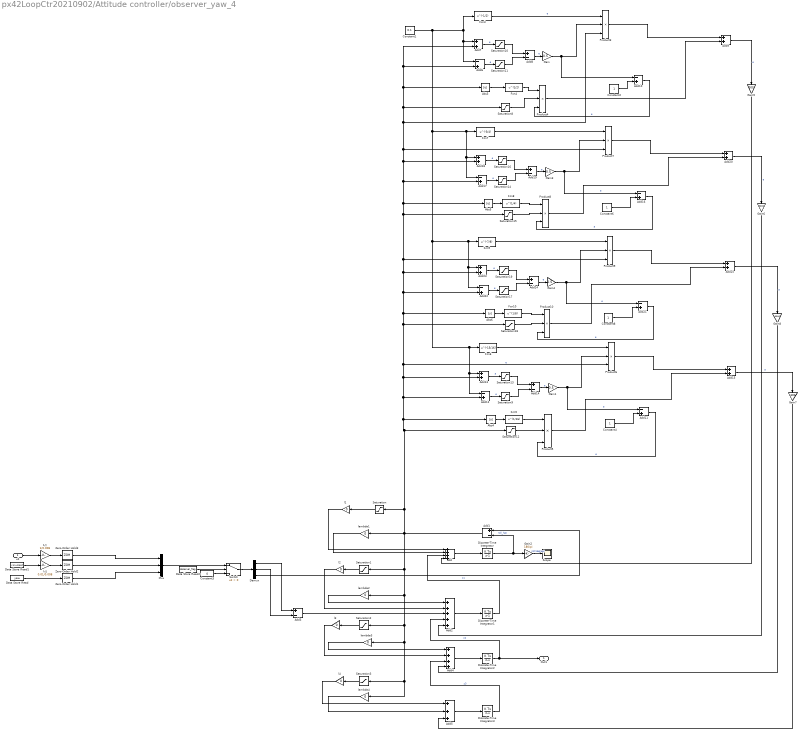
== system px42LoopCtr20210902/Attitude controller/observer_yaw_4 ==
  u2 : Inport
  1/J : Gain  Gain=1/0.008
  Abs{3..6} (4 alike) : Abs  SaturateOnIntegerOverflow=off
  Add : Sum  Inputs=++++
  Add{1,3,8,14,19,24} (6 alike) : Sum  Inputs=+-
  Add{6,10..12,16..17,21..22} (8 alike) : Sum  Inputs=-+
  Add{7,9,13,15,18,20,23,25} (8 alike) : Sum
  Add2 : Sum  Inputs=+++++
  Add4 : Sum  Inputs=++++
  Add5 : Sum  Inputs=+++
  Constant1 : Constant  Value=0.1
  Constant{2,4,6,8} (4 alike) : Constant
  Constant3 : Constant  Value=0
  Data Store Read : DataStoreRead  DataStoreName=yaw  IndexOptions=Index vector (dialog)  Indices=1  OutputSizes=1
  Data Store Read1 : DataStoreRead  DataStoreName=yaw_speed  IndexOptions=Index vector (dialog)  Indices=1  OutputSizes=1
  Data Store Read2 : DataStoreRead  DataStoreName=observer_flag  IndexOptions=Index vector (dialog)  Indices=1  OutputSizes=1
  Demux : Demux  Outputs=3
  Discrete-Time Integrator{,1..3} (4 alike) : DiscreteIntegrator  SampleTime=-1  ICPrevOutput=DiscIntNeverNeededParam  ICPrevScaledInput=DiscIntNeverNeededParam
  Fcn10 : Fcn  Expr=u^(1/8)
  Fcn3 : Fcn  Expr=u^(-1/2)
  Fcn4 : Fcn  Expr=u^(1/2)
  Fcn5 : Fcn  Expr=u^(1/16)
  Fcn6 : Fcn  Expr=u^(-15/16)
  Fcn7 : Fcn  Expr=u^(-3/4)
  Fcn8 : Fcn  Expr=u^(1/4)
  Fcn9 : Fcn  Expr=u^(-7/8)
  Gain{,1,3..4} (4 alike) : Gain  Gain=0.5
  Gain2 : Gain  Gain=180/pi
  Gain5 : Gain  Gain=300
  Gain6 : Gain  Gain=3000
  Gain7 : Gain  Gain=300
  Gain8 : Gain  Gain=5000
  Mux : Mux  Inputs=3
  Product{3..10} (8 alike) : Product  Inputs=3
  Saturation{,1..3,8..19} (16 alike) : Saturate  UpperLimit=1  LowerLimit=-1
  Scope : Scope
  Switch : Switch  Criteria=u2 > Threshold  SaturateOnIntegerOverflow=off  InputSameDT=off
  Zero-Order Hold1 : ZeroOrderHold  SampleTime=-1
  Zero-Order Hold2 : ZeroOrderHold  SampleTime=-1
  Zero-Order Hold3 : ZeroOrderHold  SampleTime=-1
  k/J : Gain  Gain=0.01/0.008
  l{1..4} (4 alike) : Gain  Gain=0
  lambda{1..4} (4 alike) : Gain  Gain=0
  Out1 : Outport
  wires:
  Data Store Read2/1 -> Switch/2
  Fcn4/1 -> Product4/1
  Fcn3/1 -> Product3/1  "e"
  Gain8/1 -> Add4/4
  Gain7/1 -> Add5/3
  Gain6/1 -> Add2/5
  Gain5/1 -> Add/4
  Add9/1 -> Gain5/1  "e"
  Add20/1 -> Gain6/1  "e"
  Add25/1 -> Gain8/1  "e"
  Add15/1 -> Gain7/1  "e"
  Saturation13/1 -> Add14/1
  Add1/1 -> Saturation1/1, lambda2/1, Saturation2/1, lambda3/1, Saturation3/1, lambda4/1, Saturation/1, Saturation15/1, Abs5/1, Add17/2, Add18/2, Abs3/1, Add7/2, Add6/2, Saturation8/1, Product3/3, Product7/3, Product9/3, Add23/2, Add22/2, Abs6/1, Saturation18/1, Product6/3, Add13/2, Add12/2, Abs4/1, Saturation12/1, lambda1/1  "e"
  Add11/1 -> Product5/3  "e"
  Add12/1 -> Saturation9/1  "e"
  Abs4/1 -> Fcn5/1
  Constant4/1 -> Add11/2
  Product6/1 -> Add15/1
  Saturation12/1 -> Product5/2
  Gain1/1 -> Product6/2, Add11/1  "e"
  Add13/1 -> Saturation13/1  "e"
  Fcn6/1 -> Product6/1
  Fcn5/1 -> Product5/1
  Saturation9/1 -> Add14/2
  Product5/1 -> Add15/2
  Constant1/1 -> Fcn9/1, Add23/1, Add22/1, Add13/1, Add12/1, Fcn6/1, Add18/1, Add17/1, Fcn7/1, Add7/1, Add6/1, Fcn3/1
  Add14/1 -> Gain1/1  "e"
  Add24/1 -> Gain4/1  "e"
  Saturation17/1 -> Add24/2
  Product10/1 -> Add25/2
  Fcn10/1 -> Product10/1
  Fcn9/1 -> Product9/1
  Add23/1 -> Saturation19/1  "e"
  Gain4/1 -> Product9/2, Add21/1  "e"
  Saturation18/1 -> Product10/2
  Saturation19/1 -> Add24/1
  Abs6/1 -> Fcn10/1
  Add21/1 -> Product10/3  "e"
  Product9/1 -> Add25/1
  Add22/1 -> Saturation17/1  "e"
  Constant8/1 -> Add21/2
  Product7/1 -> Add20/1
  Saturation15/1 -> Product8/2
  Add17/1 -> Saturation14/1  "e"
  Constant6/1 -> Add16/2
  Gain3/1 -> Product7/2, Add16/1  "e"
  Abs5/1 -> Fcn8/1
  Add16/1 -> Product8/3  "e"
  Saturation16/1 -> Add19/1
  Fcn8/1 -> Product8/1
  Fcn7/1 -> Product7/1
  Product8/1 -> Add20/2
  Add19/1 -> Gain3/1  "e"
  Saturation14/1 -> Add19/2
  Add18/1 -> Saturation16/1  "e"
  Product4/1 -> Add9/2
  Saturation11/1 -> Add8/2
  Saturation10/1 -> Add8/1
  Add10/1 -> Product4/3  "e"
  Constant2/1 -> Add10/2
  Saturation8/1 -> Product4/2
  Abs3/1 -> Fcn4/1
  Product3/1 -> Add9/1
  Gain/1 -> Product3/2, Add10/1
  Add8/1 -> Gain/1  "e"
  Add6/1 -> Saturation11/1  "e"
  Add7/1 -> Saturation10/1  "e"
  Gain2/1 -> Scope/1  "roll(degree)"
  l4/1 -> Add5/1
  lambda4/1 -> Add5/2
  Add5/1 -> Discrete-Time Integrator3/1
  Saturation3/1 -> l4/1
  l3/1 -> Add4/2
  lambda3/1 -> Add4/1
  Saturation2/1 -> l3/1
  Add4/1 -> Discrete-Time Integrator2/1
  Discrete-Time Integrator3/1 -> Add4/3  "z3"
  Add2/1 -> Discrete-Time Integrator1/1
  Add3/1 -> Add2/3
  1/J/1 -> Zero-Order Hold3/1
  u2/1 -> 1/J/1
  k/J/1 -> Zero-Order Hold2/1
  Data Store Read1/1 -> k/J/1
  l2/1 -> Add2/2
  lambda2/1 -> Add2/1
  Saturation1/1 -> l2/1
  Discrete-Time Integrator2/1 -> Add2/4, Out1/1  "z2"
  l1/1 -> Add/1
  Saturation/1 -> l1/1
  lambda1/1 -> Add/2
  Data Store Read/1 -> Zero-Order Hold1/1
  Discrete-Time Integrator/1 -> Gain2/1, Add1/2  "roll_hat"
  Discrete-Time Integrator1/1 -> Add/3  "z1"
  Add/1 -> Discrete-Time Integrator/1
  Switch/1 -> Demux/1
  Zero-Order Hold2/1 -> Mux/2
  Constant3/1 -> Switch/3
  Mux/1 -> Switch/1
  Zero-Order Hold3/1 -> Mux/1
  Demux/1 -> Add3/1
  Demux/2 -> Add3/2
  Demux/3 -> Add1/1
  Zero-Order Hold1/1 -> Mux/3

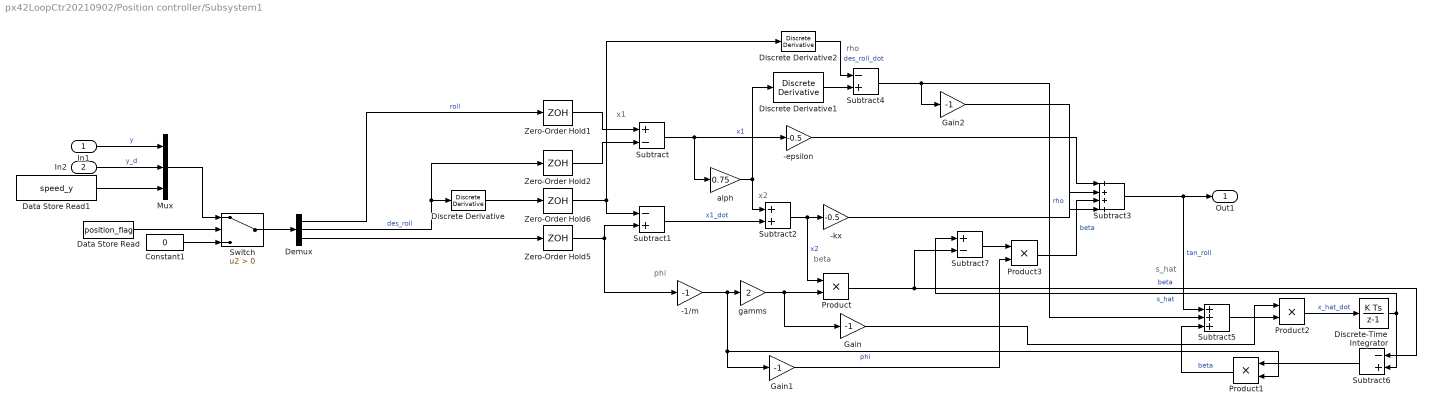
== system px42LoopCtr20210902/Position controller/Subsystem1 ==
  note: x2
  note: rho
  note: x1
  note: s_hat
  note: beta
  note: phi
  In1 : Inport
  In2 : Inport  Port=2
  -1/m : Gain  Gain=-1
  -epsilon : Gain  Gain=-0.5
  -kx : Gain  Gain=-0.5
  Constant1 : Constant  Value=0
  Data Store Read : DataStoreRead  DataStoreName=position_flag  IndexOptions=Index vector (dialog)  Indices=1  OutputSizes=1
  Data Store Read1 : DataStoreRead  DataStoreName=speed_y  IndexOptions=Index vector (dialog)  Indices=1  OutputSizes=1
  Demux : Demux  Outputs=3
  Discrete Derivative : simulink/Discrete/Discrete Derivative  gainval=1.0  ICPrevScaledInput=0.0  OutMin=[]  OutMax=[]  OutDataType=fixdt(1, 16)  OutScaling=2^-10  DoSatur=off
  Discrete Derivative1 : simulink/Discrete/Discrete Derivative  gainval=1.0  ICPrevScaledInput=0.0  OutMin=[]  OutMax=[]  OutDataType=fixdt(1, 16)  OutScaling=2^-10  DoSatur=off
  Discrete Derivative2 : simulink/Discrete/Discrete Derivative  gainval=1.0  ICPrevScaledInput=0.0  OutMin=[]  OutMax=[]  OutDataType=fixdt(1, 16)  OutScaling=2^-10  DoSatur=off
  Discrete-Time Integrator : DiscreteIntegrator  SampleTime=-1  ICPrevOutput=DiscIntNeverNeededParam  ICPrevScaledInput=DiscIntNeverNeededParam
  Gain : Gain  Gain=-1
  Gain1 : Gain  Gain=-1
  Gain2 : Gain  Gain=-1
  Mux : Mux  Inputs=3
  Product{,1..3} (4 alike) : Product
  Subtract : Sum  Inputs=+-
  Subtract1 : Sum  Inputs=-+
  Subtract2 : Sum
  Subtract3 : Sum  Inputs=++++
  Subtract4 : Sum  Inputs=-+
  Subtract5 : Sum  Inputs=+++
  Subtract6 : Sum  Inputs=-+
  Subtract7 : Sum  Inputs=+-
  Switch : Switch  Criteria=u2 > Threshold  SaturateOnIntegerOverflow=off  InputSameDT=off
  Zero-Order Hold{1..2,5..6} (4 alike) : ZeroOrderHold  SampleTime=-1
  alph : Gain  Gain=0.75
  gamms : Gain  Gain=2
  Out1 : Outport
  wires:
  Discrete Derivative/1 -> Zero-Order Hold6/1
  Demux/3 -> Zero-Order Hold5/1
  Demux/2 -> Zero-Order Hold2/1, Discrete Derivative/1  "des_roll"
  Demux/1 -> Zero-Order Hold1/1  "roll"
  Switch/1 -> Demux/1
  Data Store Read/1 -> Switch/2
  Mux/1 -> Switch/1
  In1/1 -> Mux/1  "y"
  In2/1 -> Mux/2  "y_d"
  Data Store Read1/1 -> Mux/3
  Constant1/1 -> Switch/3
  Product3/1 -> Subtract3/3  "beta"
  Subtract7/1 -> Product3/1
  Gain1/1 -> Product3/2
  Subtract5/1 -> Product2/2
  Product2/1 -> Discrete-Time Integrator/1  "x_hat_dot"
  Subtract3/1 -> Subtract5/1, Out1/1  "tan_roll"
  Discrete Derivative2/1 -> Subtract4/1  "des_roll_dot"
  Gain2/1 -> Subtract3/4
  Discrete-Time Integrator/1 -> Subtract7/1, Subtract6/2  "s_hat"
  -1/m/1 -> Gain1/1, Product1/2, gamms/1  "phi"
  Zero-Order Hold5/1 -> -1/m/1, Subtract1/2
  Subtract6/1 -> Product1/1
  Gain/1 -> Product2/1
  alph/1 -> Discrete Derivative1/1, Subtract2/1
  Subtract/1 -> alph/1, -epsilon/1  "x1"
  Product/1 -> Subtract7/2, Subtract6/1  "beta"
  Zero-Order Hold2/1 -> Subtract/2
  Zero-Order Hold1/1 -> Subtract/1
  Subtract2/1 -> Product/1, -kx/1  "x2"
  Product1/1 -> Subtract5/3  "beta"
  Subtract1/1 -> Subtract2/2  "x1_dot"
  Zero-Order Hold6/1 -> Discrete Derivative2/1, Subtract1/1
  -epsilon/1 -> Subtract3/1
  Discrete Derivative1/1 -> Subtract4/2
  gamms/1 -> Gain/1, Product/2
  Subtract4/1 -> Gain2/1, Subtract5/2  "rho"
  -kx/1 -> Subtract3/2

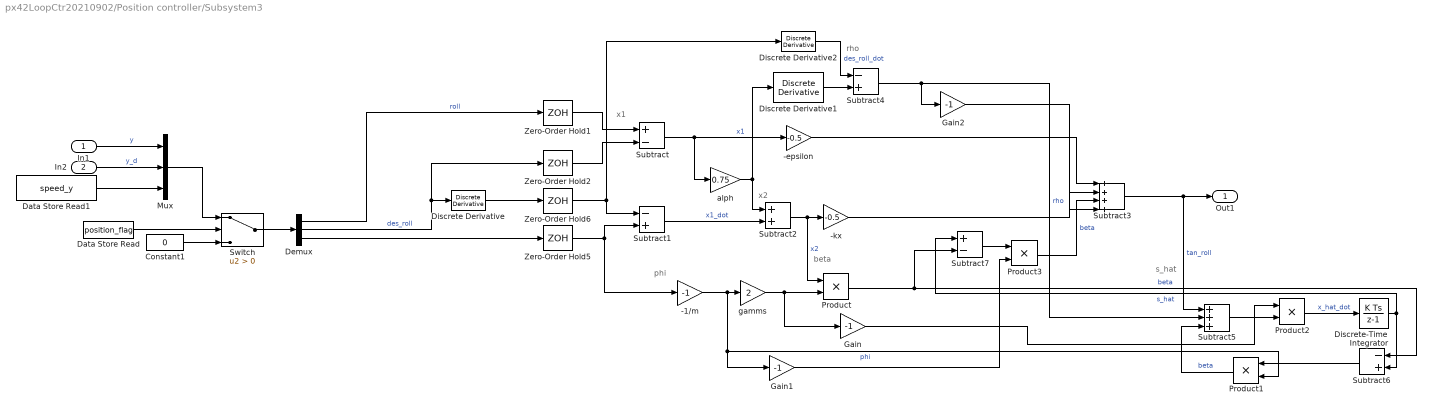
== system px42LoopCtr20210902/Position controller/Subsystem3 ==
  note: x2
  note: rho
  note: x1
  note: s_hat
  note: beta
  note: phi
  In1 : Inport
  In2 : Inport  Port=2
  -1/m : Gain  Gain=-1
  -epsilon : Gain  Gain=-0.5
  -kx : Gain  Gain=-0.5
  Constant1 : Constant  Value=0
  Data Store Read : DataStoreRead  DataStoreName=position_flag  IndexOptions=Index vector (dialog)  Indices=1  OutputSizes=1
  Data Store Read1 : DataStoreRead  DataStoreName=speed_y  IndexOptions=Index vector (dialog)  Indices=1  OutputSizes=1
  Demux : Demux  Outputs=3
  Discrete Derivative : simulink/Discrete/Discrete Derivative  gainval=1.0  ICPrevScaledInput=0.0  OutMin=[]  OutMax=[]  OutDataType=fixdt(1, 16)  OutScaling=2^-10  DoSatur=off
  Discrete Derivative1 : simulink/Discrete/Discrete Derivative  gainval=1.0  ICPrevScaledInput=0.0  OutMin=[]  OutMax=[]  OutDataType=fixdt(1, 16)  OutScaling=2^-10  DoSatur=off
  Discrete Derivative2 : simulink/Discrete/Discrete Derivative  gainval=1.0  ICPrevScaledInput=0.0  OutMin=[]  OutMax=[]  OutDataType=fixdt(1, 16)  OutScaling=2^-10  DoSatur=off
  Discrete-Time Integrator : DiscreteIntegrator  SampleTime=-1  ICPrevOutput=DiscIntNeverNeededParam  ICPrevScaledInput=DiscIntNeverNeededParam
  Gain : Gain  Gain=-1
  Gain1 : Gain  Gain=-1
  Gain2 : Gain  Gain=-1
  Mux : Mux  Inputs=3
  Product{,1..3} (4 alike) : Product
  Subtract : Sum  Inputs=+-
  Subtract1 : Sum  Inputs=-+
  Subtract2 : Sum
  Subtract3 : Sum  Inputs=++++
  Subtract4 : Sum  Inputs=-+
  Subtract5 : Sum  Inputs=+++
  Subtract6 : Sum  Inputs=-+
  Subtract7 : Sum  Inputs=+-
  Switch : Switch  Criteria=u2 > Threshold  SaturateOnIntegerOverflow=off  InputSameDT=off
  Zero-Order Hold{1..2,5..6} (4 alike) : ZeroOrderHold  SampleTime=-1
  alph : Gain  Gain=0.75
  gamms : Gain  Gain=2
  Out1 : Outport
  wires:
  Discrete Derivative/1 -> Zero-Order Hold6/1
  Demux/3 -> Zero-Order Hold5/1
  Demux/2 -> Zero-Order Hold2/1, Discrete Derivative/1  "des_roll"
  Demux/1 -> Zero-Order Hold1/1  "roll"
  Switch/1 -> Demux/1
  Data Store Read/1 -> Switch/2
  Mux/1 -> Switch/1
  In1/1 -> Mux/1  "y"
  In2/1 -> Mux/2  "y_d"
  Data Store Read1/1 -> Mux/3
  Constant1/1 -> Switch/3
  Product3/1 -> Subtract3/3  "beta"
  Subtract7/1 -> Product3/1
  Gain1/1 -> Product3/2
  Subtract5/1 -> Product2/2
  Product2/1 -> Discrete-Time Integrator/1  "x_hat_dot"
  Subtract3/1 -> Subtract5/1, Out1/1  "tan_roll"
  Discrete Derivative2/1 -> Subtract4/1  "des_roll_dot"
  Gain2/1 -> Subtract3/4
  Discrete-Time Integrator/1 -> Subtract7/1, Subtract6/2  "s_hat"
  -1/m/1 -> Gain1/1, Product1/2, gamms/1  "phi"
  Zero-Order Hold5/1 -> -1/m/1, Subtract1/2
  Subtract6/1 -> Product1/1
  Gain/1 -> Product2/1
  alph/1 -> Discrete Derivative1/1, Subtract2/1
  Subtract/1 -> alph/1, -epsilon/1  "x1"
  Product/1 -> Subtract7/2, Subtract6/1  "beta"
  Zero-Order Hold2/1 -> Subtract/2
  Zero-Order Hold1/1 -> Subtract/1
  Subtract2/1 -> Product/1, -kx/1  "x2"
  Product1/1 -> Subtract5/3  "beta"
  Subtract1/1 -> Subtract2/2  "x1_dot"
  Zero-Order Hold6/1 -> Discrete Derivative2/1, Subtract1/1
  -epsilon/1 -> Subtract3/1
  Discrete Derivative1/1 -> Subtract4/2
  gamms/1 -> Gain/1, Product/2
  Subtract4/1 -> Gain2/1, Subtract5/2  "rho"
  -kx/1 -> Subtract3/2

== system px42LoopCtr20210902/Attitude controller/Subsystem/Subsystem1 ==
  pitch : Inport
  pitch_des : Inport  Port=2
  b : Inport  Port=3
  Add : Sum  Inputs=+-
  Gain4 : Gain  Gain=-1
  Product : Product  Inputs=3
  Subsystem : Subsystem
  v* : Outport
  H : Outport  Port=2
  wires:
  Product/1 -> Gain4/1
  Gain4/1 -> v*/1
  Add/1 -> Product/1  "e"
  b/1 -> Product/3
  pitch_des/1 -> Add/2
  Subsystem/1(H) -> Product/2, H/1
  pitch/1 -> Add/1

== system px42LoopCtr20210902/Attitude controller/Subsystem1/Subsystem1 ==
  roll : Inport
  roll_des : Inport  Port=2
  b : Inport  Port=3
  Add : Sum  Inputs=+-
  Gain4 : Gain  Gain=-1
  Product : Product  Inputs=3
  Subsystem : Subsystem
  v* : Outport
  H : Outport  Port=2
  wires:
  Product/1 -> Gain4/1
  Gain4/1 -> v*/1
  Add/1 -> Product/1  "e"
  b/1 -> Product/3
  roll_des/1 -> Add/2
  Subsystem/1(H) -> H/1, Product/2
  roll/1 -> Add/1

== system px42LoopCtr20210902/Attitude controller/Subsystem6/Subsystem1 ==
  roll : Inport
  roll_des : Inport  Port=2
  b : Inport  Port=3
  Add : Sum  Inputs=+-
  Gain4 : Gain  Gain=-1
  Product : Product  Inputs=3
  Subsystem : Subsystem
  v* : Outport
  H : Outport  Port=2
  wires:
  roll/1 -> Add/1
  Subsystem/1(H) -> H/1, Product/2
  roll_des/1 -> Add/2
  b/1 -> Product/3
  Add/1 -> Product/1  "e"
  Gain4/1 -> v*/1
  Product/1 -> Gain4/1

== system px42LoopCtr20210902/Attitude controller/Subsystem7/Subsystem1 ==
  pitch : Inport
  pitch_des : Inport  Port=2
  b : Inport  Port=3
  Add : Sum  Inputs=+-
  Gain4 : Gain  Gain=-1
  Product : Product  Inputs=3
  Subsystem : Subsystem
  v* : Outport
  H : Outport  Port=2
  wires:
  pitch/1 -> Add/1
  Subsystem/1(H) -> H/1, Product/2
  pitch_des/1 -> Add/2
  b/1 -> Product/3
  Add/1 -> Product/1  "e"
  Gain4/1 -> v*/1
  Product/1 -> Gain4/1

== system px42LoopCtr20210902/Attitude controller/Subsystem/Subsystem1/Subsystem ==
  Abs : Abs  SaturateOnIntegerOverflow=off
  Add : Sum  Inputs=+-
  Add1 : Sum
  Compare To Constant1 : simulink/Logic and Bit Operations/Compare To Constant  relop=>=  const=pi/36  OutDataTypeStr=boolean
  Data Store Memory : DataStoreMemory  DataStoreName=start_time  ReadBeforeWriteMsg=warning  WriteAfterWriteMsg=warning  WriteAfterReadMsg=warning  ShowAdditionalParam=off
  Data Store Read : DataStoreRead  DataStoreName=t  IndexOptions=Index vector (dialog)  Indices=1  OutputSizes=1
  Data Store Read1 : DataStoreRead  DataStoreName=e_pitch  IndexOptions=Index vector (dialog)  Indices=1  OutputSizes=1
  Data Store Read3 : DataStoreRead  DataStoreName=start_time  IndexOptions=Index vector (dialog)  Indices=1  OutputSizes=1
  Data Store Read4 : DataStoreRead  DataStoreName=start_time  IndexOptions=Index vector (dialog)  Indices=1  OutputSizes=1
  Display : Display
  Fcn : Fcn  Expr=u(1)/(u(2)-u(3))
  MATLAB Function : MATLAB Function  TreatAsAtomicUnit=on
  Mux1 : Mux  Inputs=3
  Scope : Scope
  T : Constant  Value=5.018640350877193
  ch : Constant  Value=2
  r : Constant  Value=6.033653846153846
  start_time : Subsystem
  t : Constant  Value=0
  H : Outport
  wires:
  r/1 -> Add1/1
  Add1/1 -> H/1
  Data Store Read1/1 -> Abs/1
  Abs/1 -> Compare To Constant1/1
  T/1 -> Mux1/2
  Data Store Read/1 -> MATLAB Function/2(t), Add/1
  Add/1 -> Mux1/3
  Mux1/1 -> Fcn/1
  Data Store Read3/1 -> MATLAB Function/3(s_t), Add/2
  Data Store Read4/1 -> Display/1
  t/1 -> MATLAB Function/5(y2)
  Fcn/1 -> MATLAB Function/4(y1)
  Compare To Constant1/1 -> MATLAB Function/1(e)
  MATLAB Function/1(y) -> Add1/2, Scope/1
  ch/1 -> Mux1/1

== system px42LoopCtr20210902/Attitude controller/Subsystem1/Subsystem1/Subsystem ==
  Add1 : Sum
  Data Store Read : DataStoreRead  DataStoreName=t  IndexOptions=Index vector (dialog)  Indices=1  OutputSizes=1
  Fcn : Fcn  Expr=u(1)/(u(2)-u(3))
  Mux1 : Mux  Inputs=3
  Scope : Scope
  Switch : Switch  Threshold=5  SaturateOnIntegerOverflow=off  InputSameDT=off
  T : Constant  Value=5
  ch : Constant  Value=3
  r : Constant
  t : Constant  Value=0
  H : Outport
  wires:
  r/1 -> Add1/1
  Data Store Read/1 -> Switch/2, Mux1/3
  Mux1/1 -> Fcn/1
  ch/1 -> Mux1/1
  t/1 -> Switch/1
  T/1 -> Mux1/2
  Add1/1 -> H/1
  Fcn/1 -> Switch/3
  Switch/1 -> Scope/1, Add1/2

== system px42LoopCtr20210902/Attitude controller/Subsystem6/Subsystem1/Subsystem ==
  Abs : Abs  SaturateOnIntegerOverflow=off
  Add : Sum  Inputs=+-
  Add1 : Sum
  Compare To Constant1 : simulink/Logic and Bit Operations/Compare To Constant  relop=>=  const=pi/36  OutDataTypeStr=boolean
  Data Store Memory : DataStoreMemory  DataStoreName=start_time_roll  ReadBeforeWriteMsg=warning  WriteAfterWriteMsg=warning  WriteAfterReadMsg=warning  ShowAdditionalParam=off
  Data Store Read : DataStoreRead  DataStoreName=t  IndexOptions=Index vector (dialog)  Indices=1  OutputSizes=1
  Data Store Read1 : DataStoreRead  DataStoreName=e_pitch_roll  IndexOptions=Index vector (dialog)  Indices=1  OutputSizes=1
  Data Store Read3 : DataStoreRead  DataStoreName=start_time_roll  IndexOptions=Index vector (dialog)  Indices=1  OutputSizes=1
  Data Store Read4 : DataStoreRead  DataStoreName=start_time_roll  IndexOptions=Index vector (dialog)  Indices=1  OutputSizes=1
  Display : Display
  Fcn : Fcn  Expr=u(1)/(u(2)-u(3))
  MATLAB Function : MATLAB Function  TreatAsAtomicUnit=on
  Mux1 : Mux  Inputs=3
  Scope : Scope
  T : Constant  Value=5
  ch : Constant  Value=2
  r : Constant  Value=6.001388888888889
  start_time : Subsystem
  t : Constant  Value=0
  H : Outport
  wires:
  MATLAB Function/1(y) -> Scope/1, Add1/2
  Compare To Constant1/1 -> MATLAB Function/1(e)
  Fcn/1 -> MATLAB Function/4(y1)
  t/1 -> MATLAB Function/5(y2)
  Data Store Read4/1 -> Display/1
  Data Store Read3/1 -> Add/2, MATLAB Function/3(s_t)
  Mux1/1 -> Fcn/1
  Add/1 -> Mux1/3
  ch/1 -> Mux1/1
  Data Store Read/1 -> Add/1, MATLAB Function/2(t)
  T/1 -> Mux1/2
  Abs/1 -> Compare To Constant1/1
  Data Store Read1/1 -> Abs/1
  Add1/1 -> H/1
  r/1 -> Add1/1
